simulink model "Lab3_Step10"  (R2019b)
settings: Solver=VariableStepAuto  StartTime=0.0  StopTime=stop_time  RelTol=1e-3
InitFcn:
  | % callback_init
  | 
  | [input_wav_signal,Fs_in] = audioread('acoustic.wav');
  | 
  | %% Set Aduio Data Sample Rate
  | mp.Fs = 48000;   % sample rate of 48 kHz
  | mp.Ts = 1/mp.Fs; % sample period
  | 
  | %% Put signal into a timeseries format
  | timevals = [0:length(signal)-1]*mp.Ts;
  | input_signal = timeseries(signal,timevals);
  | 
  | %% Set the data type for audio signal (left and right channels) indata plane
  | mp.W_bits = 32;  % Word length
  | mp.F_bits = 28; % Number of fractional bits in word
  | 
  | %% Create test signals for the left and right channels
  | stop_time = length(signal) * mp.Ts;
  | 
  | %% Set the echo delay
  | delay = 1;  % delay in seconds
StopFcn:
  | y_out = output_signal.Data(:);
  | plot(y_out)
  | soundsc(y_out,mp.Fs)
settings Model: Creator=yassi  LastModifiedBy=yassi
settings DataIOCC: ReturnWorkspaceOutputs=off

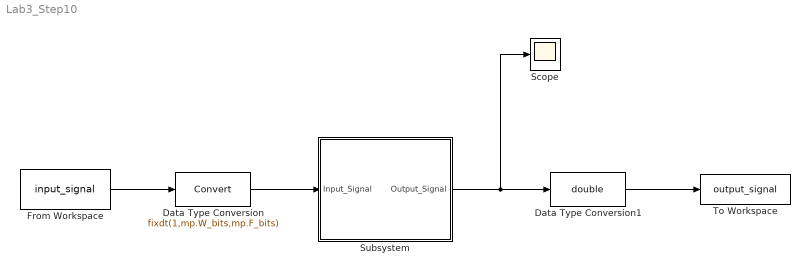
== system Lab3_Step10 ==
  Data Type Conversion : DataTypeConversion  OutDataTypeStr=fixdt(1,mp.W_bits,mp.F_bits)
  Data Type Conversion1 : DataTypeConversion  OutDataTypeStr=double
  From Workspace : FromWorkspace  VariableName=input_signal  SampleTime=mp.Ts
  Scope : Scope
  Subsystem : Subsystem
  To Workspace : ToWorkspace  VariableName=output_signal  SaveFormat=Timeseries  SampleTime=-1
  wires:
  From Workspace/1 -> Data Type Conversion/1
  Data Type Conversion/1 -> Subsystem/1(Input_Signal)
  Subsystem/1(Output_Signal) -> Data Type Conversion1/1, Scope/1
  Data Type Conversion1/1 -> To Workspace/1

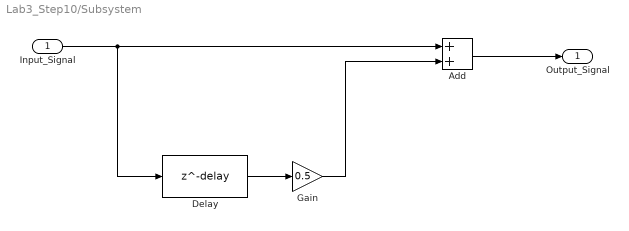
== system Lab3_Step10/Subsystem ==
  Input_Signal : Inport
  Add : Sum
  Delay : Delay  DelayLength=delay  SampleTime=mp.Ts
  Gain : Gain  Gain=0.5
  Output_Signal : Outport
  wires:
  Input_Signal/1 -> Add/1, Delay/1
  Delay/1 -> Gain/1
  Add/1 -> Output_Signal/1
  Gain/1 -> Add/2
